simulink model "uie"  (Simulink 7.9)
settings: Solver=ode45  StartTime=0.0  StopTime=10.0  RelTol=1e-3
values from neighbouring files (symbols this model uses):
  a = -1.0    (= -1)    [parameters.m]
  b = -2.0    (= -2)    [parameters.m]
  c = 0.23    [parameters.m]
  Tr = 0.04    [parameters.m]
settings Model: Creator=dede  LastModifiedBy=dede

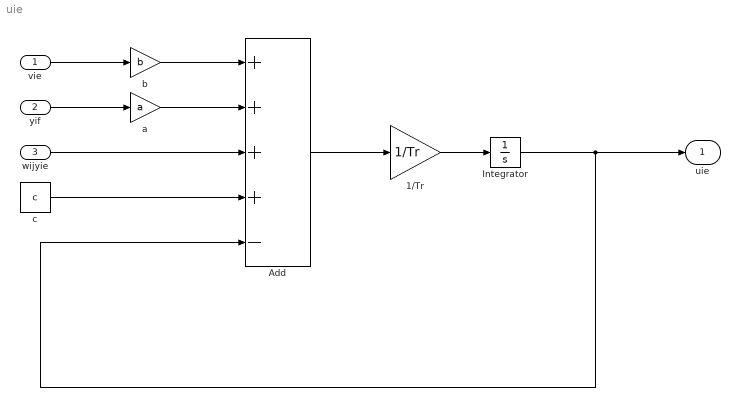
== system uie ==
  vie : Inport
  yif : Inport  Port=2
  wijyie : Inport  Port=3
  1/Tr : Gain  Gain=1/Tr
  Add : Sum  Inputs=++++-
  Integrator : Integrator
  a : Gain  Gain=a
  b : Gain  Gain=b
  c : Constant  Value=c
  uie : Outport
  wires:
  vie/1 -> b/1
  b/1 -> Add/1
  yif/1 -> a/1
  a/1 -> Add/2
  wijyie/1 -> Add/3
  c/1 -> Add/4
  Add/1 -> 1/Tr/1
  1/Tr/1 -> Integrator/1
  Integrator/1 -> Add/5, uie/1
